simulink model "chap4_4sim"  (Simulink 7.7)
settings: Solver=ode45  StartTime=0.0  StopTime=30  RelTol=1e-3
settings Model: Creator=Administrator  LastModifiedBy=ljk
settings DataIOCC: SignalLoggingName=sigsOut
settings OptimizationCC: InitFltsAndDblsToZero=on
settings DebuggingCC: SaveWithParameterizedLinksMsg=none  SignalResolutionControl=TryResolveAllWithWarning  SolverPrmCheckMsg=none  MultiTaskDSMMsg=warning  MultiTaskCondExecSysMsg=none  StrictBusMsg=Warning
settings HardwareCC: TargetUnknown=on
settings RTWCC: IncludeERTFirstTime=on
settings GRTTargetCC: TargetFcnLib=ansi_tfl_tmw.mat

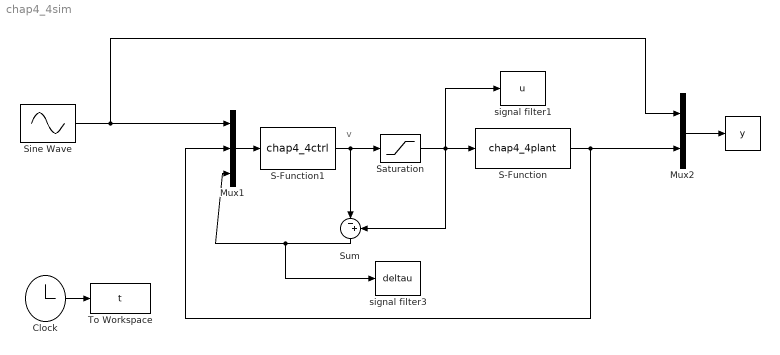
== system chap4_4sim ==
  note: v
  " " : ToWorkspace  VariableName=y  SampleTime=-1  SaveFormat=Array
  Clock : Clock
      settings: Decimation=10
  Mux1 : Mux  Inputs=3
  Mux2 : Mux  Inputs=2
  S-Function : S-Function  FunctionName=chap4_4plant  EnableBusSupport=off
  S-Function1 : S-Function  FunctionName=chap4_4ctrl  EnableBusSupport=off
  Saturation : Saturate  UpperLimit=0.3  LowerLimit=-0.3
  Sine Wave : Sin  SampleTime=0
  Sum : Sum  Inputs=|-+
  To Workspace : ToWorkspace  VariableName=t  SampleTime=-1  SaveFormat=Array
  signal filter1 : ToWorkspace  VariableName=u  SampleTime=-1  SaveFormat=Array
  signal filter3 : ToWorkspace  VariableName=deltau  SampleTime=-1  SaveFormat=Array
  wires:
  Clock/1 -> To Workspace/1
  Mux1/1 -> S-Function1/1
  Sine Wave/1 -> Mux1/1, Mux2/1
  S-Function/1 -> Mux1/2, Mux2/2
  Mux2/1 -> " "/1
  S-Function1/1 -> Sum/1, Saturation/1
  Sum/1 -> Mux1/3, signal filter3/1
  Saturation/1 -> signal filter1/1, S-Function/1, Sum/2
